simulink model "Realization_System"  (R2020b)
settings: Solver=FixedStepAuto  StartTime=0.0  StopTime=10.0  FixedStep=0.2  RelTol=1e-3
settings Model: Creator=ASUS  LastModifiedBy=ASUS
settings DataIOCC: SaveOutput=off  SaveTime=off

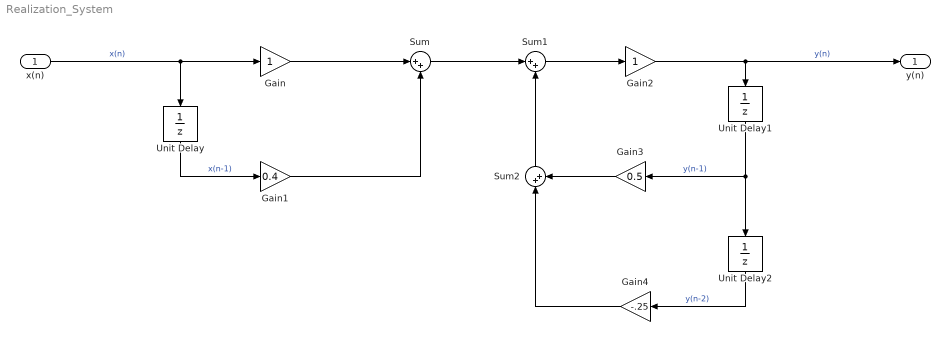
== system Realization_System ==
  x(n) : Inport  OutDataTypeStr=double  PortDimensions=1  SampleTime=[0.20000000000000001,0]
  Gain : Gain
  Gain1 : Gain  Gain=0.4
  Gain2 : Gain
  Gain3 : Gain  Gain=0.5
  Gain4 : Gain  Gain=-.25
  Sum : Sum  Inputs=|++
  Sum1 : Sum  Inputs=|++
  Sum2 : Sum  Inputs=|++
  Unit Delay : UnitDelay  SampleTime=-1  HasFrameUpgradeWarning=on
  Unit Delay1 : UnitDelay  SampleTime=-1  HasFrameUpgradeWarning=on
  Unit Delay2 : UnitDelay  SampleTime=-1  HasFrameUpgradeWarning=on
  y(n) : Outport  OutDataTypeStr=double  PortDimensions=1  SampleTime=[0.20000000000000001,0]
  wires:
  Gain2/1 -> Unit Delay1/1, y(n)/1  "y(n)"
  Gain3/1 -> Sum2/2
  Gain4/1 -> Sum2/1
  Unit Delay1/1 -> Unit Delay2/1, Gain3/1  "y(n-1)"
  Gain1/1 -> Sum/2
  Sum2/1 -> Sum1/2
  Unit Delay2/1 -> Gain4/1  "y(n-2)"
  Sum1/1 -> Gain2/1
  x(n)/1 -> Gain/1, Unit Delay/1  "x(n)"
  Gain/1 -> Sum/1
  Unit Delay/1 -> Gain1/1  "x(n-1)"
  Sum/1 -> Sum1/1
